simulink model "Prob5_MBD"  (R2020b)
settings: Solver=VariableStepAuto  StartTime=0.0  StopTime=10.0  RelTol=1e-3
InitFcn:
  | R=10;
  | C=10e-5;
settings Model: Creator=Ani  LastModifiedBy=Ani

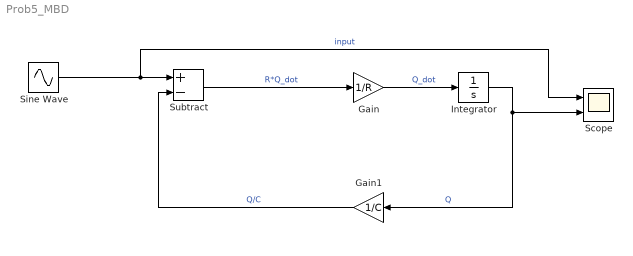
== system Prob5_MBD ==
  Gain : Gain  Gain=1/R
  Gain1 : Gain  Gain=1/C
  Integrator : Integrator
  Scope : Scope  NumInputPorts=2
  Sine Wave : Sin  Amplitude=2.5  Frequency=2  SampleTime=0
  Subtract : Sum  Inputs=+-
  wires:
  Sine Wave/1 -> Scope/1, Subtract/1  "input"
  Integrator/1 -> Scope/2, Gain1/1  "Q"
  Gain1/1 -> Subtract/2  "Q/C"
  Subtract/1 -> Gain/1  "R*Q_dot"
  Gain/1 -> Integrator/1  "Q_dot"
